simulink model "Model_turn"  (R2024a)
settings: Solver=VariableStepAuto  StartTime=0.0  StopTime=100  MaxStep=0.1  RelTol=1e-3
values from neighbouring files (symbols this model uses):
  c_SMA = 837.36    [params.m]
  Fmax_SMA = 10    [params.m]
  h_SMA = .3    (= 0.3)    [params.m]
  k_gn = m*g/0.01    (= 9810)    [contact3D_params.m]
  k_gt = m*g/0.1    (= 981)    [contact3D_params.m]
  m = 10    [contact3D_params.m]
  m_SMA = 0.0025    [params.m]
  max_SMA_Energy_J = 150    [params.m]
  mu_slide = 0.8    [contact3D_params.m]
  mu_stick = 0.9    [contact3D_params.m]
  n_segs = 10    [params.m]
  PWM_max = 0.35    [params.m]
  R_SMA = .08    (= 0.08)    [params.m]
  r_SMA2limb = 0.009    [params.m]
  swing_angle = swing_angles(i)    [params.m]
  T_amb = 23    [params.m]
  V_0 = 7    [params.m]
  v_gn_max = 0.03    [contact3D_params.m]
  v_gt_max = 0.03    [contact3D_params.m]
  vLimit = 0.01    [contact3D_params.m]
undefined symbols (not defined in the file or in its folder): Newton, Raphson, X, Y, Z
libraries: sm_lib x225, nesl_utility x185, simulink x24, simulink_extras x6
(part 1 of 16)
settings Model: SimulationMode=rapid-accelerator  Creator=lmplo  LastModifiedBy=lmplo

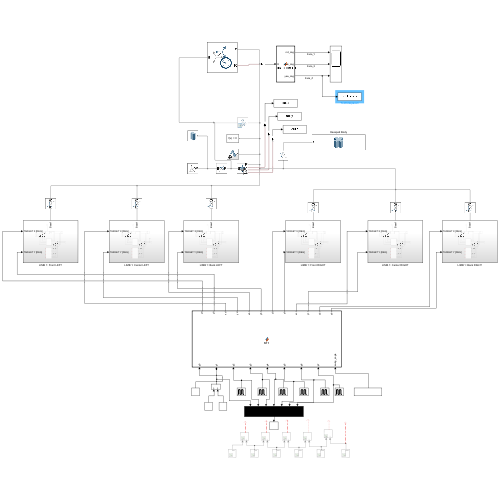
[thumbnail: Simulink's stored preview of the top-level diagram]
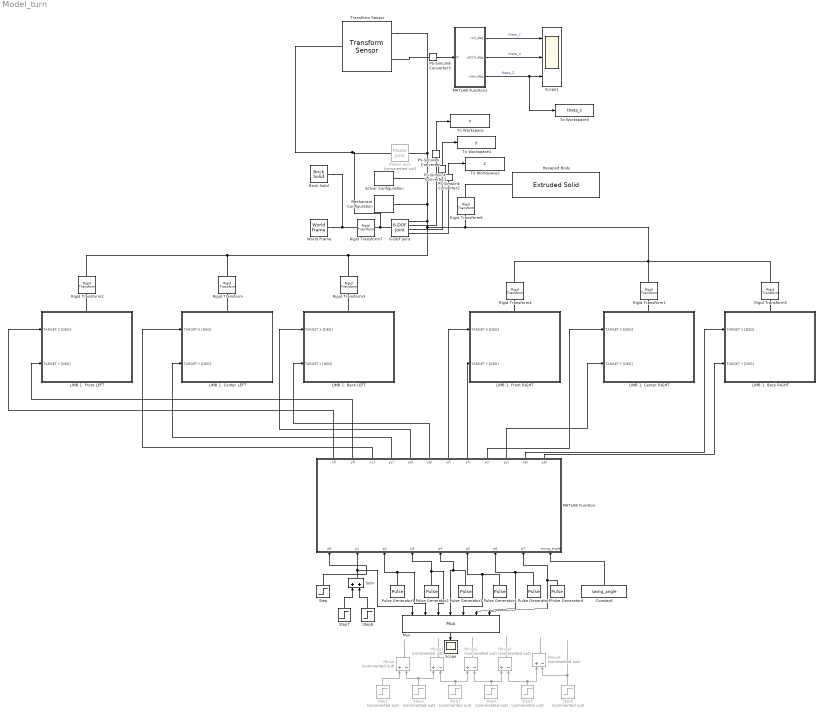
== system Model_turn ==
  6-DOF Joint : sm_lib/Joints/6-DOF Joint  JointMode=Normal  CompositeWrenchDir=FollowerOnBase  CompositeWrenchFrame=BaseFrame  SenseConstraintForce=off  SenseConstraintTorque=off  SenseTotalForce=off  SenseTotalTorque=off  PxPositionTargetSpecify=off  PxPositionTargetPriority=High  PxPositionTargetValue=0  PxPositionTargetValueUnits=m  PxVelocityTargetSpecify=off  PxVelocityTargetPriority=High  PxVelocityTargetValue=0  PxVelocityTargetValueUnits=m/s  PxEquilibriumPosition=0  PxEquilibriumPositionUnits=m  PxSpringStiffness=0  PxSpringStiffnessUnits=N/m  PxDampingCoefficient=0  PxDampingCoefficientUnits=N/(m/s)  PxLowerLimitSpecify=off  PxLowerLimitBound=-1  PxLowerLimitBoundUnits=m  PxLowerLimitStiffness=1e6  PxLowerLimitStiffnessUnits=N/m  PxLowerLimitDamping=1e3  PxLowerLimitDampingUnits=N/(m/s)  PxLowerLimitTransitionRegionWidth=1e-4  PxLowerLimitTransitionRegionWidthUnits=m  PxUpperLimitSpecify=off  PxUpperLimitBound=1  PxUpperLimitBoundUnits=m  PxUpperLimitStiffness=1e6  PxUpperLimitStiffnessUnits=N/m  PxUpperLimitDamping=1e3  PxUpperLimitDampingUnits=N/(m/s)  PxUpperLimitTransitionRegionWidth=1e-4  PxUpperLimitTransitionRegionWidthUnits=m  PxTorqueActuationMode=NoTorque  PxMotionActuationMode=ComputedMotion  PxSensePosition=on  PxSenseVelocity=off  PxSenseAcceleration=off  PxSenseTorqueForce=off  PxSenseLowerLimitTorqueForce=off  PxSenseUpperLimitTorqueForce=off  PyPositionTargetSpecify=off  PyPositionTargetPriority=High  PyPositionTargetValue=0  PyPositionTargetValueUnits=m  PyVelocityTargetSpecify=off  PyVelocityTargetPriority=High  PyVelocityTargetValue=0  PyVelocityTargetValueUnits=m/s  PyEquilibriumPosition=0  PyEquilibriumPositionUnits=m  PySpringStiffness=0  PySpringStiffnessUnits=N/m  PyDampingCoefficient=0  PyDampingCoefficientUnits=N/(m/s)  PyLowerLimitSpecify=off  PyLowerLimitBound=-1  PyLowerLimitBoundUnits=m  PyLowerLimitStiffness=1e6  PyLowerLimitStiffnessUnits=N/m  PyLowerLimitDamping=1e3  PyLowerLimitDampingUnits=N/(m/s)  PyLowerLimitTransitionRegionWidth=1e-4  PyLowerLimitTransitionRegionWidthUnits=m  PyUpperLimitSpecify=off  PyUpperLimitBound=1  PyUpperLimitBoundUnits=m  PyUpperLimitStiffness=1e6  PyUpperLimitStiffnessUnits=N/m  PyUpperLimitDamping=1e3  PyUpperLimitDampingUnits=N/(m/s)  PyUpperLimitTransitionRegionWidth=1e-4  PyUpperLimitTransitionRegionWidthUnits=m  PyTorqueActuationMode=NoTorque  PyMotionActuationMode=ComputedMotion  PySensePosition=on  PySenseVelocity=off  PySenseAcceleration=off  PySenseTorqueForce=off  PySenseLowerLimitTorqueForce=off  PySenseUpperLimitTorqueForce=off  PzPositionTargetSpecify=off  PzPositionTargetPriority=High  PzPositionTargetValue=0  PzPositionTargetValueUnits=m  PzVelocityTargetSpecify=off  PzVelocityTargetPriority=High  PzVelocityTargetValue=0  PzVelocityTargetValueUnits=m/s  PzEquilibriumPosition=0  PzEquilibriumPositionUnits=m  PzSpringStiffness=0  PzSpringStiffnessUnits=N/m  PzDampingCoefficient=0  PzDampingCoefficientUnits=N/(m/s)  PzLowerLimitSpecify=off  PzLowerLimitBound=-1  PzLowerLimitBoundUnits=m  PzLowerLimitStiffness=1e6  PzLowerLimitStiffnessUnits=N/m  PzLowerLimitDamping=1e3  PzLowerLimitDampingUnits=N/(m/s)  PzLowerLimitTransitionRegionWidth=1e-4  PzLowerLimitTransitionRegionWidthUnits=m  PzUpperLimitSpecify=off  PzUpperLimitBound=1  PzUpperLimitBoundUnits=m  PzUpperLimitStiffness=1e6  PzUpperLimitStiffnessUnits=N/m  PzUpperLimitDamping=1e3  PzUpperLimitDampingUnits=N/(m/s)  PzUpperLimitTransitionRegionWidth=1e-4  PzUpperLimitTransitionRegionWidthUnits=m  PzTorqueActuationMode=NoTorque  PzMotionActuationMode=ComputedMotion  PzSensePosition=on  PzSenseVelocity=off  PzSenseAcceleration=off  PzSenseTorqueForce=off  PzSenseLowerLimitTorqueForce=off  PzSenseUpperLimitTorqueForce=off  SphPositionTargetSpecify=off  SphPositionTargetPriority=High  SphPositionTargetRotationMethod=None  SphPositionTargetFollAlignAxisA=+X  SphPositionTargetBaseAlignAxisA=+Y  SphPositionTargetFollAlignAxisB=+Y  SphPositionTargetBaseAlignAxisB=+Z  SphPositionTargetRotationStandardAxis=+Z  SphPositionTargetRotationAngle=0  SphPositionTargetRotationAngleUnits=deg  SphPositionTargetRotationArbitraryAxis=[0 0 1]  SphPositionTargetRotationSequenceAxes=FollowerAxes  SphPositionTargetRotationSequence=XYX  SphPositionTargetRotationSequenceAngles=[0 0 0]  SphPositionTargetRotationSequenceAnglesUnits=deg  SphPositionTargetRotationMatrix=[1 0 0;0 1 0;0 0 1]  SphPositionTargetQuaternion=[1 0 0 0]  SphVelocityTargetSpecify=off  SphVelocityTargetPriority=High  SphVelocityTargetValue=[0 0 0]  SphVelocityTargetValueUnits=deg/s  SphVelocityTargetInFollowerFrame=on  SphEqPosRotationMethod=None  SphEqPosFollAlignAxisA=+X  SphEqPosBaseAlignAxisA=+Y  SphEqPosFollAlignAxisB=+Y  SphEqPosBaseAlignAxisB=+Z  SphEqPosRotationStandardAxis=+Z  SphEqPosRotationAngle=0  SphEqPosRotationAngleUnits=deg  SphEqPosRotationArbitraryAxis=[0 0 1]  SphEqPosRotationSequenceAxes=FollowerAxes  SphEqPosRotationSequence=XYX  SphEqPosRotationSequenceAngles=[0 0 0]  SphEqPosRotationSequenceAnglesUnits=deg  SphEqPosRotationMatrix=[1 0 0;0 1 0;0 0 1]  SphEqPosQuaternion=[1 0 0 0]  SphSpringStiffness=0  SphSpringStiffnessUnits=N*m/deg  SphDampingCoefficient=0  SphDampingCoefficientUnits=N*m/(deg/s)  SphLowerLimitSpecify=off  SphLowerLimitBound=15  SphLowerLimitBoundUnits=deg  SphLowerLimitStiffness=1e4  SphLowerLimitStiffnessUnits=N*m/deg  SphLowerLimitDamping=10  SphLowerLimitDampingUnits=N*m/(deg/s)  SphLowerLimitTransitionRegionWidth=0.1  SphLowerLimitTransitionRegionWidthUnits=deg  SphUpperLimitSpecify=off  SphUpperLimitBound=45  SphUpperLimitBoundUnits=deg  SphUpperLimitStiffness=1e4  SphUpperLimitStiffnessUnits=N*m/deg  SphUpperLimitDamping=10  SphUpperLimitDampingUnits=N*m/(deg/s)  SphUpperLimitTransitionRegionWidth=0.1  SphUpperLimitTransitionRegionWidthUnits=deg  SphTorqueActuationMode=NoTorque  SphActuateTorqueX=off  SphActuateTorqueY=off  SphActuateTorqueZ=off  SphActuateTorque=off  SphActuationFrame=BaseFrame  SphSensePosition=off  SphSenseVelocityX=off  SphSenseVelocityY=off  SphSenseVelocityZ=off  SphSenseVelocity=off  SphSenseAccelerationX=off  SphSenseAccelerationY=off  SphSenseAccelerationZ=off  SphSenseAcceleration=off  SphSenseLowerLimitTorqueMag=off  SphSenseUpperLimitTorqueMag=off  SphSensingFrame=BaseFrame
  Brick Solid : sm_lib/Body Elements/Brick Solid  BrickDimensions=[10 10 0.001]  BrickDimensionsUnits=m  ExportEntireGeometry=off  InertiaType=CalculateFromGeometry  BasedOnType=Density  Density=1000  DensityUnits=kg/m^3  Mass=1  MassUnits=kg  CenterOfMass=[0 0 0]  CenterOfMassUnits=m  MomentsOfInertia=[1 1 1]  MomentsOfInertiaUnits=kg*m^2  ProductsOfInertia=[0 0 0]  ProductsOfInertiaUnits=kg*m^2  GraphicType=FromGeometry  MarkerShape=Sphere  MarkerSize=10  GraphicVisPropType=SimpleVisualProperties  GraphicDiffuseColor=[0.4 0.2 0.0]  GraphicOpacity=1  GraphicSpecularColor=[0.5 0.5 0.5 1.0]  GraphicAmbientColor=[0.15 0.15 0.15 1.0]  GraphicEmissiveColor=[0.0 0.0 0.0 1.0]  GraphicShininess=75  DoExposeReferenceFrame=on  SerializedFrames=<Frames/>
  Constant : Constant  Value=swing_angle
  Hexapod Body : sm_lib/Body Elements/Extruded Solid  ExtrusionType=General  PolygonNumSides=6  PolygonOuterRadius=.1  PolygonOuterRadiusUnits=m  ExportEntireGeometry=off  ExtrusionCrossSection=[-.1 0; -.05 -.07; .05 -.07; .1 0; .05 .07; -.05 .07]  ExtrusionCrossSectionUnits=m  ExportConvexHullGeometry=off  ExtrusionLength=.05  ExtrusionLengthUnits=m  InertiaType=CalculateFromGeometry  BasedOnType=Density  Density=10  DensityUnits=kg/m^3  Mass=1  MassUnits=kg  CenterOfMass=[0 0 0]  CenterOfMassUnits=m  MomentsOfInertia=[1 1 1]  MomentsOfInertiaUnits=kg*m^2  ProductsOfInertia=[0 0 0]  ProductsOfInertiaUnits=kg*m^2  GraphicType=FromGeometry  MarkerShape=Sphere  MarkerSize=10  GraphicVisPropType=SimpleVisualProperties  GraphicDiffuseColor=[0.5 0.5 0.5]  GraphicOpacity=1  GraphicSpecularColor=[0.5 0.5 0.5 1.0]  GraphicAmbientColor=[0.15 0.15 0.15 1.0]  GraphicEmissiveColor=[0.0 0.0 0.0 1.0]  GraphicShininess=75  DoExposeReferenceFrame=on  SerializedFrames=<Frames/>
  LIMB 1: Back LEFT : Subsystem
      settings: PortSchema="{\"entries\":[{\"content\":{\"sides\":[{\"content\":{\"connectorIds\":[\"In1\",\"In2\"]},\"type\":\"ConnectorPlacement.EquallySpacedRectSide\",\"uuid\":\"dac3a422-23dc-41de-9456-f1b703ee7ea4\"},{\"content\":{\"side\":\"RIGHT\"},\"type\":\"ConnectorPlacement.EquallySpacedRectSide\",\"uuid\":\"acd4b41e-2563-470e-afc8-f7cd5e457540\"},{\"content\":{\"connectorIds\":[\"LConn1\"],\"side\":\"TOP\"},\"type\":\"ConnectorPlacement.EquallySpacedRectSide\",\"uuid\":\"2403ebe1-3ea7-4eb6-be2b-197ca3d8e68e\"}]},\"type\":\"ConnectorPlacement.EquallySpacedConnector\",\"uuid\":\"537b2e86-94c9-41ef-b748-fab54b193b4a\"}],\"packageUris\":[\"http://schema.mathworks.com/mf0/Connector/R2020b\"],\"version\":\"1.0\"}"
  LIMB 1: Back RIGHT : Subsystem
      settings: PortSchema="{\"entries\":[{\"content\":{\"sides\":[{\"content\":{\"connectorIds\":[\"In1\",\"In2\"]},\"type\":\"ConnectorPlacement.EquallySpacedRectSide\",\"uuid\":\"dac3a422-23dc-41de-9456-f1b703ee7ea4\"},{\"content\":{\"side\":\"RIGHT\"},\"type\":\"ConnectorPlacement.EquallySpacedRectSide\",\"uuid\":\"acd4b41e-2563-470e-afc8-f7cd5e457540\"},{\"content\":{\"connectorIds\":[\"LConn1\"],\"side\":\"TOP\"},\"type\":\"ConnectorPlacement.EquallySpacedRectSide\",\"uuid\":\"2403ebe1-3ea7-4eb6-be2b-197ca3d8e68e\"}]},\"type\":\"ConnectorPlacement.EquallySpacedConnector\",\"uuid\":\"537b2e86-94c9-41ef-b748-fab54b193b4a\"}],\"packageUris\":[\"http://schema.mathworks.com/mf0/Connector/R2020b\"],\"version\":\"1.0\"}"
  LIMB 1: Center LEFT : Subsystem
      settings: PortSchema="{\"entries\":[{\"content\":{\"sides\":[{\"content\":{\"connectorIds\":[\"In1\",\"In2\"]},\"type\":\"ConnectorPlacement.EquallySpacedRectSide\",\"uuid\":\"dac3a422-23dc-41de-9456-f1b703ee7ea4\"},{\"content\":{\"side\":\"RIGHT\"},\"type\":\"ConnectorPlacement.EquallySpacedRectSide\",\"uuid\":\"acd4b41e-2563-470e-afc8-f7cd5e457540\"},{\"content\":{\"connectorIds\":[\"LConn1\"],\"side\":\"TOP\"},\"type\":\"ConnectorPlacement.EquallySpacedRectSide\",\"uuid\":\"2403ebe1-3ea7-4eb6-be2b-197ca3d8e68e\"}]},\"type\":\"ConnectorPlacement.EquallySpacedConnector\",\"uuid\":\"537b2e86-94c9-41ef-b748-fab54b193b4a\"}],\"packageUris\":[\"http://schema.mathworks.com/mf0/Connector/R2020b\"],\"version\":\"1.0\"}"
  LIMB 1: Center RIGHT : Subsystem
      settings: PortSchema="{\"entries\":[{\"content\":{\"sides\":[{\"content\":{\"connectorIds\":[\"In1\",\"In2\"]},\"type\":\"ConnectorPlacement.EquallySpacedRectSide\",\"uuid\":\"dac3a422-23dc-41de-9456-f1b703ee7ea4\"},{\"content\":{\"side\":\"RIGHT\"},\"type\":\"ConnectorPlacement.EquallySpacedRectSide\",\"uuid\":\"acd4b41e-2563-470e-afc8-f7cd5e457540\"},{\"content\":{\"connectorIds\":[\"LConn1\"],\"side\":\"TOP\"},\"type\":\"ConnectorPlacement.EquallySpacedRectSide\",\"uuid\":\"2403ebe1-3ea7-4eb6-be2b-197ca3d8e68e\"}]},\"type\":\"ConnectorPlacement.EquallySpacedConnector\",\"uuid\":\"537b2e86-94c9-41ef-b748-fab54b193b4a\"}],\"packageUris\":[\"http://schema.mathworks.com/mf0/Connector/R2020b\"],\"version\":\"1.0\"}"
  LIMB 1: Front LEFT : Subsystem
      settings: PortSchema="{\"entries\":[{\"content\":{\"sides\":[{\"content\":{\"connectorIds\":[\"In1\",\"In2\"]},\"type\":\"ConnectorPlacement.EquallySpacedRectSide\",\"uuid\":\"dac3a422-23dc-41de-9456-f1b703ee7ea4\"},{\"content\":{\"side\":\"RIGHT\"},\"type\":\"ConnectorPlacement.EquallySpacedRectSide\",\"uuid\":\"acd4b41e-2563-470e-afc8-f7cd5e457540\"},{\"content\":{\"connectorIds\":[\"LConn1\"],\"side\":\"TOP\"},\"type\":\"ConnectorPlacement.EquallySpacedRectSide\",\"uuid\":\"2403ebe1-3ea7-4eb6-be2b-197ca3d8e68e\"}]},\"type\":\"ConnectorPlacement.EquallySpacedConnector\",\"uuid\":\"537b2e86-94c9-41ef-b748-fab54b193b4a\"}],\"packageUris\":[\"http://schema.mathworks.com/mf0/Connector/R2020b\"],\"version\":\"1.0\"}"
  LIMB 1: Front RIGHT : Subsystem
      settings: PortSchema="{\"entries\":[{\"content\":{\"sides\":[{\"content\":{\"connectorIds\":[\"In1\",\"In2\"]},\"type\":\"ConnectorPlacement.EquallySpacedRectSide\",\"uuid\":\"dac3a422-23dc-41de-9456-f1b703ee7ea4\"},{\"content\":{\"side\":\"RIGHT\"},\"type\":\"ConnectorPlacement.EquallySpacedRectSide\",\"uuid\":\"acd4b41e-2563-470e-afc8-f7cd5e457540\"},{\"content\":{\"connectorIds\":[\"LConn1\"],\"side\":\"TOP\"},\"type\":\"ConnectorPlacement.EquallySpacedRectSide\",\"uuid\":\"2403ebe1-3ea7-4eb6-be2b-197ca3d8e68e\"}]},\"type\":\"ConnectorPlacement.EquallySpacedConnector\",\"uuid\":\"537b2e86-94c9-41ef-b748-fab54b193b4a\"}],\"packageUris\":[\"http://schema.mathworks.com/mf0/Connector/R2020b\"],\"version\":\"1.0\"}"
  MATLAB Function : MATLAB Function  TreatAsAtomicUnit=on
  MATLAB Function1 : MATLAB Function  TreatAsAtomicUnit=on
  Mechanism Configuration : sm_lib/Utilities/Mechanism Configuration  UniformGravity=Constant  GravityVector=[0 0 -9.80665]  GravityVectorUnits=m/s^2  LinearizationDelta=0.001  JointModeTransitionNonlinearIterations=2
  Minus{,1..4} (5 alike) : Sum  Commented=on  Inputs=+-
  Mux : Mux  Inputs=7
  PS-Simulink Converter{,1..3} (4 alike) : nesl_utility/PS-Simulink Converter  PhysicalDomain=network_engine_domain  SubClassName=ps_output  LeftPortType=input  RightPortType=output  PseudoPeriodic=off  Frequencies=[]  VectorFormat=inherit  Unit=inherit  AffineConversion=off
  Planar Joint : sm_lib/Joints/Planar Joint  Commented=on  JointMode=Normal  CompositeWrenchDir=FollowerOnBase  CompositeWrenchFrame=BaseFrame  SenseConstraintForce=off  SenseConstraintTorque=off  SenseTotalForce=off  SenseTotalTorque=off  PxPositionTargetSpecify=off  PxPositionTargetPriority=High  PxPositionTargetValue=0  PxPositionTargetValueUnits=m  PxVelocityTargetSpecify=off  PxVelocityTargetPriority=High  PxVelocityTargetValue=0  PxVelocityTargetValueUnits=m/s  PxEquilibriumPosition=0  PxEquilibriumPositionUnits=m  PxSpringStiffness=0  PxSpringStiffnessUnits=N/m  PxDampingCoefficient=0  PxDampingCoefficientUnits=N/(m/s)  PxLowerLimitSpecify=off  PxLowerLimitBound=-1  PxLowerLimitBoundUnits=m  PxLowerLimitStiffness=1e6  PxLowerLimitStiffnessUnits=N/m  PxLowerLimitDamping=1e3  PxLowerLimitDampingUnits=N/(m/s)  PxLowerLimitTransitionRegionWidth=1e-4  PxLowerLimitTransitionRegionWidthUnits=m  PxUpperLimitSpecify=off  PxUpperLimitBound=1  PxUpperLimitBoundUnits=m  PxUpperLimitStiffness=1e6  PxUpperLimitStiffnessUnits=N/m  PxUpperLimitDamping=1e3  PxUpperLimitDampingUnits=N/(m/s)  PxUpperLimitTransitionRegionWidth=1e-4  PxUpperLimitTransitionRegionWidthUnits=m  PxTorqueActuationMode=NoTorque  PxMotionActuationMode=ComputedMotion  PxSensePosition=off  PxSenseVelocity=off  PxSenseAcceleration=off  PxSenseTorqueForce=off  PxSenseLowerLimitTorqueForce=off  PxSenseUpperLimitTorqueForce=off  PyPositionTargetSpecify=off  PyPositionTargetPriority=High  PyPositionTargetValue=0  PyPositionTargetValueUnits=m  PyVelocityTargetSpecify=off  PyVelocityTargetPriority=High  PyVelocityTargetValue=0  PyVelocityTargetValueUnits=m/s  PyEquilibriumPosition=0  PyEquilibriumPositionUnits=m  PySpringStiffness=0  PySpringStiffnessUnits=N/m  PyDampingCoefficient=0  PyDampingCoefficientUnits=N/(m/s)  PyLowerLimitSpecify=off  PyLowerLimitBound=-1  PyLowerLimitBoundUnits=m  PyLowerLimitStiffness=1e6  PyLowerLimitStiffnessUnits=N/m  PyLowerLimitDamping=1e3  PyLowerLimitDampingUnits=N/(m/s)  PyLowerLimitTransitionRegionWidth=1e-4  PyLowerLimitTransitionRegionWidthUnits=m  PyUpperLimitSpecify=off  PyUpperLimitBound=1  PyUpperLimitBoundUnits=m  PyUpperLimitStiffness=1e6  PyUpperLimitStiffnessUnits=N/m  PyUpperLimitDamping=1e3  PyUpperLimitDampingUnits=N/(m/s)  PyUpperLimitTransitionRegionWidth=1e-4  PyUpperLimitTransitionRegionWidthUnits=m  PyTorqueActuationMode=NoTorque  PyMotionActuationMode=ComputedMotion  PySensePosition=off  PySenseVelocity=off  PySenseAcceleration=off  PySenseTorqueForce=off  PySenseLowerLimitTorqueForce=off  PySenseUpperLimitTorqueForce=off  RzPositionTargetSpecify=off  RzPositionTargetPriority=High  RzPositionTargetValue=0  RzPositionTargetValueUnits=deg  RzVelocityTargetSpecify=off  RzVelocityTargetPriority=High  RzVelocityTargetValue=0  RzVelocityTargetValueUnits=deg/s  RzEquilibriumPosition=0  RzEquilibriumPositionUnits=deg  RzSpringStiffness=0  RzSpringStiffnessUnits=N*m/deg  RzDampingCoefficient=0  RzDampingCoefficientUnits=N*m/(deg/s)  RzLowerLimitSpecify=off  RzLowerLimitBound=-90  RzLowerLimitBoundUnits=deg  RzLowerLimitStiffness=1e4  RzLowerLimitStiffnessUnits=N*m/deg  RzLowerLimitDamping=10  RzLowerLimitDampingUnits=N*m/(deg/s)  RzLowerLimitTransitionRegionWidth=0.1  RzLowerLimitTransitionRegionWidthUnits=deg  RzUpperLimitSpecify=off  RzUpperLimitBound=90  RzUpperLimitBoundUnits=deg  RzUpperLimitStiffness=1e4  RzUpperLimitStiffnessUnits=N*m/deg  RzUpperLimitDamping=10  RzUpperLimitDampingUnits=N*m/(deg/s)  RzUpperLimitTransitionRegionWidth=0.1  RzUpperLimitTransitionRegionWidthUnits=deg  RzTorqueActuationMode=NoTorque  RzMotionActuationMode=ComputedMotion  RzSensePosition=off  RzSenseVelocity=off  RzSenseAcceleration=off  RzSenseTorqueForce=off  RzSenseLowerLimitTorqueForce=off  RzSenseUpperLimitTorqueForce=off
  Pulse Generator1 : DiscretePulseGenerator  PulseType=Time based  Period=30  PulseWidth=16  PhaseDelay=10
  Pulse Generator2 : DiscretePulseGenerator  PulseType=Time based  Period=30  PulseWidth=16  PhaseDelay=15
  Pulse Generator3 : DiscretePulseGenerator  PulseType=Time based  Period=30  PulseWidth=16  PhaseDelay=20
  Pulse Generator4 : DiscretePulseGenerator  PulseType=Time based  Period=30  PulseWidth=16  PhaseDelay=25
  Pulse Generator5 : DiscretePulseGenerator  PulseType=Time based  Period=30  PulseWidth=16  PhaseDelay=30
  Pulse Generator6 : DiscretePulseGenerator  PulseType=Time based  Period=30  PulseWidth=16  PhaseDelay=35
  Rigid Transform : sm_lib/Frames and Transforms/Rigid Transform  RotationMethod=StandardAxis  FollAlignAxisA=+X  BaseAlignAxisA=+Y  FollAlignAxisB=+Y  BaseAlignAxisB=+Z  RotationStandardAxis=+Y  RotationAngle=30  RotationAngleUnits=deg  RotationArbitraryAxis=[0 0 1]  RotationSequenceAxes=FollowerAxes  RotationSequence=XYX  RotationSequenceAngles=[0 0 0]  RotationSequenceAnglesUnits=deg  RotationMatrix=[1 0 0;0 1 0;0 0 1]  Quaternion=[1 0 0 0]  TranslationMethod=Cartesian  TranslationCartesianOffset=[-0.1 0 0]  TranslationCartesianOffsetUnits=m  TranslationStandardAxis=+Z  TranslationStandardOffset=0  TranslationStandardOffsetUnits=m  TranslationROffset=0  TranslationROffsetUnits=m  TranslationThetaOffset=0  TranslationThetaOffsetUnits=deg  TranslationZOffset=0  TranslationZOffsetUnits=m
  Rigid Transform1 : sm_lib/Frames and Transforms/Rigid Transform  RotationMethod=StandardAxis  FollAlignAxisA=+X  BaseAlignAxisA=+Y  FollAlignAxisB=+Y  BaseAlignAxisB=+Z  RotationStandardAxis=+Y  RotationAngle=-30  RotationAngleUnits=deg  RotationArbitraryAxis=[0 0 1]  RotationSequenceAxes=FollowerAxes  RotationSequence=XYX  RotationSequenceAngles=[0 0 0]  RotationSequenceAnglesUnits=deg  RotationMatrix=[1 0 0;0 1 0;0 0 1]  Quaternion=[1 0 0 0]  TranslationMethod=Cartesian  TranslationCartesianOffset=[0.1 0 0]  TranslationCartesianOffsetUnits=m  TranslationStandardAxis=+Z  TranslationStandardOffset=0  TranslationStandardOffsetUnits=m  TranslationROffset=0  TranslationROffsetUnits=m  TranslationThetaOffset=0  TranslationThetaOffsetUnits=deg  TranslationZOffset=0  TranslationZOffsetUnits=m
  Rigid Transform2 : sm_lib/Frames and Transforms/Rigid Transform  RotationMethod=StandardAxis  FollAlignAxisA=+X  BaseAlignAxisA=+Y  FollAlignAxisB=+Y  BaseAlignAxisB=+Z  RotationStandardAxis=+Y  RotationAngle=30  RotationAngleUnits=deg  RotationArbitraryAxis=[0 0 1]  RotationSequenceAxes=BaseAxes  RotationSequence=XYZ  RotationSequenceAngles=[0 0 0]  RotationSequenceAnglesUnits=deg  RotationMatrix=[1 0 0;0 1 0;0 0 1]  Quaternion=[1 0 0 0]  TranslationMethod=Cartesian  TranslationCartesianOffset=[-0.05 0.07 0]  TranslationCartesianOffsetUnits=m  TranslationStandardAxis=+Z  TranslationStandardOffset=0  TranslationStandardOffsetUnits=m  TranslationROffset=0  TranslationROffsetUnits=m  TranslationThetaOffset=0  TranslationThetaOffsetUnits=deg  TranslationZOffset=0  TranslationZOffsetUnits=m
  Rigid Transform3 : sm_lib/Frames and Transforms/Rigid Transform  RotationMethod=StandardAxis  FollAlignAxisA=+X  BaseAlignAxisA=+Y  FollAlignAxisB=+Y  BaseAlignAxisB=+Z  RotationStandardAxis=+Y  RotationAngle=30  RotationAngleUnits=deg  RotationArbitraryAxis=[0 0 1]  RotationSequenceAxes=FollowerAxes  RotationSequence=XYX  RotationSequenceAngles=[0 0 0]  RotationSequenceAnglesUnits=deg  RotationMatrix=[1 0 0;0 1 0;0 0 1]  Quaternion=[1 0 0 0]  TranslationMethod=Cartesian  TranslationCartesianOffset=[-0.05 -0.07 0]  TranslationCartesianOffsetUnits=m  TranslationStandardAxis=+Z  TranslationStandardOffset=0  TranslationStandardOffsetUnits=m  TranslationROffset=0  TranslationROffsetUnits=m  TranslationThetaOffset=0  TranslationThetaOffsetUnits=deg  TranslationZOffset=0  TranslationZOffsetUnits=m
  Rigid Transform4 : sm_lib/Frames and Transforms/Rigid Transform  RotationMethod=StandardAxis  FollAlignAxisA=+X  BaseAlignAxisA=+Y  FollAlignAxisB=+Y  BaseAlignAxisB=+Z  RotationStandardAxis=+Y  RotationAngle=-30  RotationAngleUnits=deg  RotationArbitraryAxis=[0 0 1]  RotationSequenceAxes=BaseAxes  RotationSequence=XYZ  RotationSequenceAngles=[0 0 0]  RotationSequenceAnglesUnits=deg  RotationMatrix=[1 0 0;0 1 0;0 0 1]  Quaternion=[1 0 0 0]  TranslationMethod=Cartesian  TranslationCartesianOffset=[0.05 0.07 0]  TranslationCartesianOffsetUnits=m  TranslationStandardAxis=+Z  TranslationStandardOffset=0  TranslationStandardOffsetUnits=m  TranslationROffset=0  TranslationROffsetUnits=m  TranslationThetaOffset=0  TranslationThetaOffsetUnits=deg  TranslationZOffset=0  TranslationZOffsetUnits=m
  Rigid Transform5 : sm_lib/Frames and Transforms/Rigid Transform  RotationMethod=StandardAxis  FollAlignAxisA=+X  BaseAlignAxisA=+Y  FollAlignAxisB=+Y  BaseAlignAxisB=+Z  RotationStandardAxis=+Y  RotationAngle=-30  RotationAngleUnits=deg  RotationArbitraryAxis=[0 0 1]  RotationSequenceAxes=FollowerAxes  RotationSequence=XYX  RotationSequenceAngles=[0 0 0]  RotationSequenceAnglesUnits=deg  RotationMatrix=[1 0 0;0 1 0;0 0 1]  Quaternion=[1 0 0 0]  TranslationMethod=Cartesian  TranslationCartesianOffset=[0.05 -0.07 0]  TranslationCartesianOffsetUnits=m  TranslationStandardAxis=+Z  TranslationStandardOffset=0  TranslationStandardOffsetUnits=m  TranslationROffset=0  TranslationROffsetUnits=m  TranslationThetaOffset=0  TranslationThetaOffsetUnits=deg  TranslationZOffset=0  TranslationZOffsetUnits=m
  Rigid Transform6 : sm_lib/Frames and Transforms/Rigid Transform  RotationMethod=None  FollAlignAxisA=+X  BaseAlignAxisA=+Y  FollAlignAxisB=+Y  BaseAlignAxisB=+Z  RotationStandardAxis=+Z  RotationAngle=0  RotationAngleUnits=deg  RotationArbitraryAxis=[0 0 1]  RotationSequenceAxes=FollowerAxes  RotationSequence=XYX  RotationSequenceAngles=[0 0 0]  RotationSequenceAnglesUnits=deg  RotationMatrix=[1 0 0;0 1 0;0 0 1]  Quaternion=[1 0 0 0]  TranslationMethod=Cartesian  TranslationCartesianOffset=[0 0 0.02]  TranslationCartesianOffsetUnits=m  TranslationStandardAxis=+Z  TranslationStandardOffset=0  TranslationStandardOffsetUnits=m  TranslationROffset=0  TranslationROffsetUnits=m  TranslationThetaOffset=0  TranslationThetaOffsetUnits=deg  TranslationZOffset=0  TranslationZOffsetUnits=m
  Rigid Transform7 : sm_lib/Frames and Transforms/Rigid Transform  RotationMethod=StandardAxis  FollAlignAxisA=+X  BaseAlignAxisA=+Y  FollAlignAxisB=+Y  BaseAlignAxisB=+Z  RotationStandardAxis=+Y  RotationAngle=0  RotationAngleUnits=deg  RotationArbitraryAxis=[0 0 1]  RotationSequenceAxes=FollowerAxes  RotationSequence=XYX  RotationSequenceAngles=[0 0 0]  RotationSequenceAnglesUnits=deg  RotationMatrix=[1 0 0;0 1 0;0 0 1]  Quaternion=[1 0 0 0]  TranslationMethod=Cartesian  TranslationCartesianOffset=[0 0 0.87]  TranslationCartesianOffsetUnits=m  TranslationStandardAxis=+Z  TranslationStandardOffset=0  TranslationStandardOffsetUnits=m  TranslationROffset=0  TranslationROffsetUnits=m  TranslationThetaOffset=0  TranslationThetaOffsetUnits=deg  TranslationZOffset=0  TranslationZOffsetUnits=m
  Scope : Scope
  Scope1 : Scope  NumInputPorts=3
  Solver Configuration : nesl_utility/Solver Configuration  PhysicalDomain=network_engine_domain  SubClassName=solver  LeftPortType=input  RightPortType=generic  Tones=[]  Harmonics=[]  SimulateNoise=off  Profile=off  UseLocalSampling=off  EnableSwitchedLinearOptims=on  FrequencyDomain=off  UseCCode=off  RelTol=0.001  AbsTol=0.001  MinStep=1e-09  ToWorkspace=off  RevertToSquareIcSolve=off  NumHomotopyIterations=100  PhasorMode=off  PhasorModeNumHarmonics=1  ConsistencySolver=NEWTON_XTOL_AFTER_FTOL  IndexReductionMethod=DerivativeReplacement  DoDC=off  ResidualTolerance=1e-09  ConsistencyTolSource=GLOBAL  ConsistencyAbsTol=0.001  ConsistencyRelTol=0.001  ConsistencyTolFactor=0.001  UseLocalSolver=off  LocalSolverChoice=NE_BACKWARD_EULER_ADVANCER  ResolveIndetEquations=on  FunctionEvalNumThread=1  LocalSolverSampleTime=0.001  DoFixedCost=off  MaxNonlinIter=3  MaxModeIter=2  ComputeImpulses=off  ImpulseIterations=2  LinearAlgebra=auto  LinearAlgebraNumThread=0  EquationFormulation=NE_TIME_EF  DelaysMemoryBudget=1024  AutomaticFiltering=on  FilteringTimeConstant=0.001  PartitionStorageMethod=AS_NEEDED  PartitionMemoryBudget=1024  PartitionMethod=ROBUST  MultibodyUseLocalSolver=off  MultibodyLocalSolverChoice=ODE1  MultibodyLocalSolverSampleTime=0.001
  Step : Step  Time=5  Before=1  After=0  SampleTime=0
  Step1 : Step  Commented=on  Time=5  SampleTime=0
  Step2 : Step  Commented=on  Time=10  SampleTime=0
  Step3 : Step  Commented=on  Time=15  SampleTime=0
  Step4 : Step  Commented=on  Time=20  SampleTime=0
  Step5 : Step  Commented=on  Time=25  SampleTime=0
  Step6 : Step  Commented=on  Time=30  SampleTime=0
  Step7 : Step  Time=5  SampleTime=0
  Step8 : Step  Time=10  After=-1  SampleTime=0
  Sum : Sum
  To Workspace : ToWorkspace  VariableName=x  SaveFormat=Timeseries  SampleTime=-1
  To Workspace1 : ToWorkspace  VariableName=y  SaveFormat=Timeseries  SampleTime=-1
  To Workspace2 : ToWorkspace  VariableName=z  SaveFormat=Timeseries  SampleTime=-1
  To Workspace3 : ToWorkspace  VariableName=theta_z  SaveFormat=Timeseries  SampleTime=-1
  Transform Sensor : sm_lib/Frames and Transforms/Transform Sensor  MeasurementFrame=NonRotatingBase  RotationSequence=XYZ  SenseAngle=off  SenseAxis=off  SenseQ=off  SenseR=on  SenseRotationSequence=off  SenseOmegaX=off  SenseOmegaY=off  SenseOmegaZ=off  SenseOmega=off  SenseQDot=off  SenseRDot=off  SenseRotationSequenceDot=off  SenseAlphaX=off  SenseAlphaY=off  SenseAlphaZ=off  SenseAlpha=off  SenseQDDot=off  SenseRDDot=off  SenseX=off  SenseY=off  SenseZ=off  SenseXYZ=off  SenseRad=off  SenseAzim=off  SenseDist=off  SenseInc=off  SenseXDot=off  SenseYDot=off  SenseZDot=off  SenseXYZDot=off  SenseRadDot=off  SenseAzimDot=off  SenseDistDot=off  SenseIncDot=off  SenseXDDot=off  SenseYDDot=off  SenseZDDot=off  SenseXYZDDot=off  SenseRadDDot=off  SenseAzimDDot=off  SenseDistDDot=off  SenseIncDDot=off
  World Frame : sm_lib/Frames and Transforms/World Frame
  wires:
  MATLAB Function/1(xfl) -> LIMB 1: Front LEFT/1(TARGET X [DEG])
  MATLAB Function/2(yfl) -> LIMB 1: Front LEFT/2(TARGET Y [DEG])
  MATLAB Function/3(xcl) -> LIMB 1: Center LEFT/1(TARGET X [DEG])
  MATLAB Function/4(ycl) -> LIMB 1: Center LEFT/2(TARGET Y [DEG])
  MATLAB Function/5(xbl) -> LIMB 1: Back LEFT/1(TARGET X [DEG])
  MATLAB Function/6(ybl) -> LIMB 1: Back LEFT/2(TARGET Y [DEG])
  MATLAB Function/7(xfr) -> LIMB 1: Front RIGHT/1(TARGET X [DEG])
  MATLAB Function/8(yfr) -> LIMB 1: Front RIGHT/2(TARGET Y [DEG])
  MATLAB Function/9(xcr) -> LIMB 1: Center RIGHT/1(TARGET X [DEG])
  MATLAB Function/10(ycr) -> LIMB 1: Center RIGHT/2(TARGET Y [DEG])
  MATLAB Function/11(xbr) -> LIMB 1: Back RIGHT/1(TARGET X [DEG])
  MATLAB Function/12(ybr) -> LIMB 1: Back RIGHT/2(TARGET Y [DEG])
  Step4/1 -> Minus3/1, Minus2/2
  Minus/1 -> ?
  Step1/1 -> Minus/1
  Step2/1 -> Minus1/1, Minus/2
  Minus1/1 -> ?
  Step3/1 -> Minus2/1, Minus1/2
  Minus2/1 -> ?
  Step/1 -> MATLAB Function/1(p0)
  Minus3/1 -> ?
  Step5/1 -> Minus3/2, Minus4/1
  Minus4/1 -> ?
  Step6/1 -> Minus4/2
  Pulse Generator1/1 -> Mux/2, MATLAB Function/3(p2)
  Pulse Generator2/1 -> Mux/3, MATLAB Function/4(p3)
  Pulse Generator3/1 -> Mux/4, MATLAB Function/5(p4)
  Pulse Generator4/1 -> Mux/5, MATLAB Function/6(p5)
  Pulse Generator5/1 -> Mux/6, MATLAB Function/7(p6)
  Mux/1 -> Scope/1
  Pulse Generator6/1 -> Mux/7, MATLAB Function/8(p7)
  Sum/1 -> Mux/1, MATLAB Function/2(p1)
  Step7/1 -> Sum/1
  Step8/1 -> Sum/2
  Constant/1 -> MATLAB Function/9(swing_angle)
  PS-Simulink Converter/1 -> To Workspace/1
  PS-Simulink Converter1/1 -> To Workspace1/1
  PS-Simulink Converter2/1 -> To Workspace2/1
  MATLAB Function1/2(pitch_deg) -> Scope1/2  "theta_X"
  PS-Simulink Converter3/1 -> MATLAB Function1/1(R)
  MATLAB Function1/3(yaw_deg) -> To Workspace3/1, Scope1/3  "theta_Z"
  MATLAB Function1/1(roll_deg) -> Scope1/1  "theta_Y"
  connections:
  Rigid Transform/RConn1 -- LIMB 1: Center LEFT/LConn1
  Rigid Transform2/RConn1 -- LIMB 1: Front LEFT/LConn1
  Rigid Transform3/RConn1 -- LIMB 1: Back LEFT/LConn1
  Planar Joint/RConn1 -- Transform Sensor/RConn1 -- Solver Configuration/RConn1 -- Mechanism Configuration/RConn1 -- Rigid Transform5/LConn1 -- Rigid Transform1/LConn1 -- Rigid Transform4/LConn1 -- Rigid Transform6/LConn1 -- Rigid Transform2/LConn1 -- Rigid Transform/LConn1 -- Rigid Transform3/LConn1 -- 6-DOF Joint/RConn1
  Rigid Transform5/RConn1 -- LIMB 1: Back RIGHT/LConn1
  Rigid Transform1/RConn1 -- LIMB 1: Center RIGHT/LConn1
  Rigid Transform4/RConn1 -- LIMB 1: Front RIGHT/LConn1
  Hexapod Body/RConn1 -- Rigid Transform6/RConn1
  World Frame/RConn1 -- Brick Solid/RConn1 -- Rigid Transform7/LConn1
  Rigid Transform7/RConn1 -- Planar Joint/LConn1 -- Transform Sensor/LConn1 -- 6-DOF Joint/LConn1
  6-DOF Joint/RConn2 -- PS-Simulink Converter/LConn1
  6-DOF Joint/RConn3 -- PS-Simulink Converter1/LConn1
  6-DOF Joint/RConn4 -- PS-Simulink Converter2/LConn1
  PS-Simulink Converter3/LConn1 -- Transform Sensor/RConn2

== system Model_turn/LIMB 1: Back LEFT ==
  TARGET X [DEG] : Inport
  TARGET Y [DEG] : Inport  Port=2
  BANG-BANG CONTROLLER : MATLAB Function  TreatAsAtomicUnit=on
  Constant : Constant  Value=PWM_max
  "DUTY CYCLE " : Scope  NumInputPorts=4
  Derivative : Derivative
  Derivative1 : Derivative
  Integrator : Integrator
  Integrator1 : Integrator
  Limb 1 : Subsystem
      settings: PortSchema="{\"entries\":[{\"content\":{\"sides\":[{\"content\":{\"connectorIds\":[\"In1\",\"In2\",\"In3\",\"In4\"]},\"type\":\"ConnectorPlacement.EquallySpacedRectSide\",\"uuid\":\"1cfbebb6-90a9-4503-841a-11205e4f7b86\"},{\"content\":{\"connectorIds\":[\"Out1\",\"Out2\",\"Out3\",\"Out4\",\"Out5\",\"Out6\"],\"side\":\"RIGHT\"},\"type\":\"ConnectorPlacement.EquallySpacedRectSide\",\"uuid\":\"1fe5f3cc-98d4-4c2f-97d4-d32079cd1e1f\"},{\"content\":{\"connectorIds\":[\"LConn1\"],\"side\":\"TOP\"},\"type\":\"ConnectorPlacement.EquallySpacedRectSide\",\"uuid\":\"8adc0629-c4c5-41e3-bf7c-2c474717e53c\"}]},\"type\":\"ConnectorPlacement.EquallySpacedConnector\",\"uuid\":\"10590026-c19e-4697-bf09-c537692c54fc\"}],\"packageUris\":[\"http://schema.mathworks.com/mf0/Connector/R2020b\"],\"version\":\"1.0\"}"
  PID CONTROLLER : MATLAB Function  TreatAsAtomicUnit=on
  POSITION : Scope  NumInputPorts=2
  Scope : Scope
  Sum : Sum  Inputs=|+-
  Sum1 : Sum  Inputs=|+-
  [0, 1]{,1..3} (4 alike) : Saturate  UpperLimit=1  LowerLimit=0
  Base1 : PMIOPort  Side=Left
  wires:
  PID CONTROLLER/4(D4) -> ?
  PID CONTROLLER/2(D2) -> ?
  "[0, 1]2"/1 -> Limb 1/2(Duty Cycle 3), "DUTY CYCLE "/3
  PID CONTROLLER/3(D3) -> ?
  Derivative/1 -> PID CONTROLLER/2(deX)
  TARGET X [DEG]/1 -> Sum1/1, BANG-BANG CONTROLLER/3(Target_X)
  PID CONTROLLER/1(D1) -> ?
  Integrator/1 -> PID CONTROLLER/3(seX)
  TARGET Y [DEG]/1 -> BANG-BANG CONTROLLER/4(Target_Y), Sum/1
  Sum/1 -> PID CONTROLLER/4(eY), Derivative1/1, Integrator1/1
  BANG-BANG CONTROLLER/2(D2) -> "[0, 1]1"/1
  Limb 1/1(theta_X) -> POSITION/1, Sum1/2, BANG-BANG CONTROLLER/1(theta_X)
  BANG-BANG CONTROLLER/1(D1) -> "[0, 1]"/1
  "[0, 1]"/1 -> "DUTY CYCLE "/1, Limb 1/4(Duty Cycle 1)
  Derivative1/1 -> PID CONTROLLER/5(deY)
  BANG-BANG CONTROLLER/4(D4) -> "[0, 1]3"/1
  Integrator1/1 -> PID CONTROLLER/6(seY)
  Constant/1 -> BANG-BANG CONTROLLER/5(PWM_max), PID CONTROLLER/7(PWM_max)
  "[0, 1]1"/1 -> "DUTY CYCLE "/2, Limb 1/3(Duty Cycle 2)
  Sum1/1 -> PID CONTROLLER/1(eX), Scope/1, Derivative/1, Integrator/1
  "[0, 1]3"/1 -> "DUTY CYCLE "/4, Limb 1/1(Duty Cycle 4)
  BANG-BANG CONTROLLER/3(D3) -> "[0, 1]2"/1
  Limb 1/2(theta_Y) -> POSITION/2, Sum/2, BANG-BANG CONTROLLER/2(theta_Y)
  connections:
  Base1/RConn1 -- Limb 1/LConn1

== system Model_turn/LIMB 1: Back RIGHT ==
  TARGET X [DEG] : Inport
  TARGET Y [DEG] : Inport  Port=2
  BANG-BANG CONTROLLER : MATLAB Function  TreatAsAtomicUnit=on
  Constant : Constant  Value=PWM_max
  "DUTY CYCLE " : Scope  NumInputPorts=4
  Derivative : Derivative
  Derivative1 : Derivative
  Integrator : Integrator
  Integrator1 : Integrator
  Limb 1 : Subsystem
      settings: PortSchema="{\"entries\":[{\"content\":{\"sides\":[{\"content\":{\"connectorIds\":[\"In1\",\"In2\",\"In3\",\"In4\"]},\"type\":\"ConnectorPlacement.EquallySpacedRectSide\",\"uuid\":\"1cfbebb6-90a9-4503-841a-11205e4f7b86\"},{\"content\":{\"connectorIds\":[\"Out1\",\"Out2\",\"Out3\",\"Out4\",\"Out5\",\"Out6\"],\"side\":\"RIGHT\"},\"type\":\"ConnectorPlacement.EquallySpacedRectSide\",\"uuid\":\"1fe5f3cc-98d4-4c2f-97d4-d32079cd1e1f\"},{\"content\":{\"connectorIds\":[\"LConn1\"],\"side\":\"TOP\"},\"type\":\"ConnectorPlacement.EquallySpacedRectSide\",\"uuid\":\"8adc0629-c4c5-41e3-bf7c-2c474717e53c\"}]},\"type\":\"ConnectorPlacement.EquallySpacedConnector\",\"uuid\":\"10590026-c19e-4697-bf09-c537692c54fc\"}],\"packageUris\":[\"http://schema.mathworks.com/mf0/Connector/R2020b\"],\"version\":\"1.0\"}"
  PID CONTROLLER : MATLAB Function  TreatAsAtomicUnit=on
  POSITION : Scope  NumInputPorts=2
  Scope : Scope
  Sum : Sum  Inputs=|+-
  Sum1 : Sum  Inputs=|+-
  [0, 1]{,1..3} (4 alike) : Saturate  UpperLimit=1  LowerLimit=0
  Base1 : PMIOPort  Side=Left
  wires:
  Limb 1/2(theta_Y) -> BANG-BANG CONTROLLER/2(theta_Y), Sum/2, POSITION/2
  BANG-BANG CONTROLLER/3(D3) -> "[0, 1]2"/1
  "[0, 1]3"/1 -> Limb 1/1(Duty Cycle 4), "DUTY CYCLE "/4
  Sum1/1 -> Integrator/1, Derivative/1, Scope/1, PID CONTROLLER/1(eX)
  "[0, 1]1"/1 -> Limb 1/3(Duty Cycle 2), "DUTY CYCLE "/2
  Constant/1 -> PID CONTROLLER/7(PWM_max), BANG-BANG CONTROLLER/5(PWM_max)
  Integrator1/1 -> PID CONTROLLER/6(seY)
  BANG-BANG CONTROLLER/4(D4) -> "[0, 1]3"/1
  Derivative1/1 -> PID CONTROLLER/5(deY)
  "[0, 1]"/1 -> Limb 1/4(Duty Cycle 1), "DUTY CYCLE "/1
  BANG-BANG CONTROLLER/1(D1) -> "[0, 1]"/1
  Limb 1/1(theta_X) -> BANG-BANG CONTROLLER/1(theta_X), Sum1/2, POSITION/1
  BANG-BANG CONTROLLER/2(D2) -> "[0, 1]1"/1
  Sum/1 -> Integrator1/1, Derivative1/1, PID CONTROLLER/4(eY)
  TARGET Y [DEG]/1 -> Sum/1, BANG-BANG CONTROLLER/4(Target_Y)
  Integrator/1 -> PID CONTROLLER/3(seX)
  PID CONTROLLER/1(D1) -> ?
  TARGET X [DEG]/1 -> BANG-BANG CONTROLLER/3(Target_X), Sum1/1
  Derivative/1 -> PID CONTROLLER/2(deX)
  PID CONTROLLER/3(D3) -> ?
  "[0, 1]2"/1 -> "DUTY CYCLE "/3, Limb 1/2(Duty Cycle 3)
  PID CONTROLLER/2(D2) -> ?
  PID CONTROLLER/4(D4) -> ?
  connections:
  Base1/RConn1 -- Limb 1/LConn1

== system Model_turn/LIMB 1: Center LEFT ==
  TARGET X [DEG] : Inport
  TARGET Y [DEG] : Inport  Port=2
  BANG-BANG CONTROLLER : MATLAB Function  TreatAsAtomicUnit=on
  Constant : Constant  Value=PWM_max
  "DUTY CYCLE " : Scope  NumInputPorts=4
  Derivative : Derivative
  Derivative1 : Derivative
  Integrator : Integrator
  Integrator1 : Integrator
  Limb 1 : Subsystem
      settings: PortSchema="{\"entries\":[{\"content\":{\"sides\":[{\"content\":{\"connectorIds\":[\"In1\",\"In2\",\"In3\",\"In4\"]},\"type\":\"ConnectorPlacement.EquallySpacedRectSide\",\"uuid\":\"1cfbebb6-90a9-4503-841a-11205e4f7b86\"},{\"content\":{\"connectorIds\":[\"Out1\",\"Out2\",\"Out3\",\"Out4\",\"Out5\",\"Out6\"],\"side\":\"RIGHT\"},\"type\":\"ConnectorPlacement.EquallySpacedRectSide\",\"uuid\":\"1fe5f3cc-98d4-4c2f-97d4-d32079cd1e1f\"},{\"content\":{\"connectorIds\":[\"LConn1\"],\"side\":\"TOP\"},\"type\":\"ConnectorPlacement.EquallySpacedRectSide\",\"uuid\":\"8adc0629-c4c5-41e3-bf7c-2c474717e53c\"}]},\"type\":\"ConnectorPlacement.EquallySpacedConnector\",\"uuid\":\"10590026-c19e-4697-bf09-c537692c54fc\"}],\"packageUris\":[\"http://schema.mathworks.com/mf0/Connector/R2020b\"],\"version\":\"1.0\"}"
  PID CONTROLLER : MATLAB Function  TreatAsAtomicUnit=on
  POSITION : Scope  NumInputPorts=2
  Scope : Scope
  Scope1 : Scope
  Sum : Sum  Inputs=|+-
  Sum1 : Sum  Inputs=|+-
  [0, 1]{,1..3} (4 alike) : Saturate  UpperLimit=1  LowerLimit=0
  Base1 : PMIOPort  Side=Left
  wires:
  Limb 1/2(theta_Y) -> BANG-BANG CONTROLLER/2(theta_Y), Sum/2, POSITION/2
  BANG-BANG CONTROLLER/3(D3) -> "[0, 1]2"/1
  "[0, 1]3"/1 -> Limb 1/1(Duty Cycle 4), "DUTY CYCLE "/4
  Sum1/1 -> Integrator/1, Derivative/1, Scope/1, PID CONTROLLER/1(eX)
  "[0, 1]1"/1 -> Limb 1/3(Duty Cycle 2), "DUTY CYCLE "/2
  Constant/1 -> PID CONTROLLER/7(PWM_max), BANG-BANG CONTROLLER/5(PWM_max)
  Integrator1/1 -> PID CONTROLLER/6(seY)
  BANG-BANG CONTROLLER/4(D4) -> "[0, 1]3"/1
  Derivative1/1 -> PID CONTROLLER/5(deY)
  "[0, 1]"/1 -> Limb 1/4(Duty Cycle 1), "DUTY CYCLE "/1
  BANG-BANG CONTROLLER/1(D1) -> "[0, 1]"/1
  Limb 1/1(theta_X) -> BANG-BANG CONTROLLER/1(theta_X), Sum1/2, POSITION/1
  BANG-BANG CONTROLLER/2(D2) -> "[0, 1]1"/1
  Sum/1 -> Integrator1/1, Derivative1/1, PID CONTROLLER/4(eY)
  TARGET Y [DEG]/1 -> Scope1/1, Sum/1, BANG-BANG CONTROLLER/4(Target_Y)
  Integrator/1 -> PID CONTROLLER/3(seX)
  PID CONTROLLER/1(D1) -> ?
  TARGET X [DEG]/1 -> BANG-BANG CONTROLLER/3(Target_X), Sum1/1
  Derivative/1 -> PID CONTROLLER/2(deX)
  PID CONTROLLER/3(D3) -> ?
  "[0, 1]2"/1 -> "DUTY CYCLE "/3, Limb 1/2(Duty Cycle 3)
  PID CONTROLLER/2(D2) -> ?
  PID CONTROLLER/4(D4) -> ?
  connections:
  Base1/RConn1 -- Limb 1/LConn1

== system Model_turn/LIMB 1: Center RIGHT ==
  TARGET X [DEG] : Inport
  TARGET Y [DEG] : Inport  Port=2
  BANG-BANG CONTROLLER : MATLAB Function  TreatAsAtomicUnit=on
  Constant : Constant  Value=PWM_max
  "DUTY CYCLE " : Scope  NumInputPorts=4
  Derivative : Derivative
  Derivative1 : Derivative
  Integrator : Integrator
  Integrator1 : Integrator
  Limb 1 : Subsystem
      settings: PortSchema="{\"entries\":[{\"content\":{\"sides\":[{\"content\":{\"connectorIds\":[\"In1\",\"In2\",\"In3\",\"In4\"]},\"type\":\"ConnectorPlacement.EquallySpacedRectSide\",\"uuid\":\"1cfbebb6-90a9-4503-841a-11205e4f7b86\"},{\"content\":{\"connectorIds\":[\"Out1\",\"Out2\",\"Out3\",\"Out4\",\"Out5\",\"Out6\"],\"side\":\"RIGHT\"},\"type\":\"ConnectorPlacement.EquallySpacedRectSide\",\"uuid\":\"1fe5f3cc-98d4-4c2f-97d4-d32079cd1e1f\"},{\"content\":{\"connectorIds\":[\"LConn1\"],\"side\":\"TOP\"},\"type\":\"ConnectorPlacement.EquallySpacedRectSide\",\"uuid\":\"8adc0629-c4c5-41e3-bf7c-2c474717e53c\"}]},\"type\":\"ConnectorPlacement.EquallySpacedConnector\",\"uuid\":\"10590026-c19e-4697-bf09-c537692c54fc\"}],\"packageUris\":[\"http://schema.mathworks.com/mf0/Connector/R2020b\"],\"version\":\"1.0\"}"
  PID CONTROLLER : MATLAB Function  TreatAsAtomicUnit=on
  POSITION : Scope  NumInputPorts=2
  Scope : Scope
  Sum : Sum  Inputs=|+-
  Sum1 : Sum  Inputs=|+-
  [0, 1]{,1..3} (4 alike) : Saturate  UpperLimit=1  LowerLimit=0
  Base1 : PMIOPort  Side=Left
  wires:
  PID CONTROLLER/4(D4) -> ?
  PID CONTROLLER/2(D2) -> ?
  "[0, 1]2"/1 -> Limb 1/2(Duty Cycle 3), "DUTY CYCLE "/3
  PID CONTROLLER/3(D3) -> ?
  Derivative/1 -> PID CONTROLLER/2(deX)
  TARGET X [DEG]/1 -> Sum1/1, BANG-BANG CONTROLLER/3(Target_X)
  PID CONTROLLER/1(D1) -> ?
  Integrator/1 -> PID CONTROLLER/3(seX)
  TARGET Y [DEG]/1 -> BANG-BANG CONTROLLER/4(Target_Y), Sum/1
  Sum/1 -> PID CONTROLLER/4(eY), Derivative1/1, Integrator1/1
  BANG-BANG CONTROLLER/2(D2) -> "[0, 1]1"/1
  Limb 1/1(theta_X) -> POSITION/1, Sum1/2, BANG-BANG CONTROLLER/1(theta_X)
  BANG-BANG CONTROLLER/1(D1) -> "[0, 1]"/1
  "[0, 1]"/1 -> "DUTY CYCLE "/1, Limb 1/4(Duty Cycle 1)
  Derivative1/1 -> PID CONTROLLER/5(deY)
  BANG-BANG CONTROLLER/4(D4) -> "[0, 1]3"/1
  Integrator1/1 -> PID CONTROLLER/6(seY)
  Constant/1 -> BANG-BANG CONTROLLER/5(PWM_max), PID CONTROLLER/7(PWM_max)
  "[0, 1]1"/1 -> "DUTY CYCLE "/2, Limb 1/3(Duty Cycle 2)
  Sum1/1 -> PID CONTROLLER/1(eX), Scope/1, Derivative/1, Integrator/1
  "[0, 1]3"/1 -> "DUTY CYCLE "/4, Limb 1/1(Duty Cycle 4)
  BANG-BANG CONTROLLER/3(D3) -> "[0, 1]2"/1
  Limb 1/2(theta_Y) -> POSITION/2, Sum/2, BANG-BANG CONTROLLER/2(theta_Y)
  connections:
  Base1/RConn1 -- Limb 1/LConn1

== system Model_turn/LIMB 1: Front LEFT ==
  TARGET X [DEG] : Inport
  TARGET Y [DEG] : Inport  Port=2
  BANG-BANG CONTROLLER : MATLAB Function  TreatAsAtomicUnit=on
  Constant : Constant  Value=PWM_max
  "DUTY CYCLE " : Scope  NumInputPorts=4
  Derivative : Derivative
  Derivative1 : Derivative
  Integrator : Integrator
  Integrator1 : Integrator
  Limb 1 : Subsystem
      settings: PortSchema="{\"entries\":[{\"content\":{\"sides\":[{\"content\":{\"connectorIds\":[\"In1\",\"In2\",\"In3\",\"In4\"]},\"type\":\"ConnectorPlacement.EquallySpacedRectSide\",\"uuid\":\"1cfbebb6-90a9-4503-841a-11205e4f7b86\"},{\"content\":{\"connectorIds\":[\"Out1\",\"Out2\",\"Out3\",\"Out4\",\"Out5\",\"Out6\"],\"side\":\"RIGHT\"},\"type\":\"ConnectorPlacement.EquallySpacedRectSide\",\"uuid\":\"1fe5f3cc-98d4-4c2f-97d4-d32079cd1e1f\"},{\"content\":{\"connectorIds\":[\"LConn1\"],\"side\":\"TOP\"},\"type\":\"ConnectorPlacement.EquallySpacedRectSide\",\"uuid\":\"8adc0629-c4c5-41e3-bf7c-2c474717e53c\"}]},\"type\":\"ConnectorPlacement.EquallySpacedConnector\",\"uuid\":\"10590026-c19e-4697-bf09-c537692c54fc\"}],\"packageUris\":[\"http://schema.mathworks.com/mf0/Connector/R2020b\"],\"version\":\"1.0\"}"
  PID CONTROLLER : MATLAB Function  TreatAsAtomicUnit=on
  POSITION : Scope  NumInputPorts=2
  Scope : Scope
  Scope1 : Scope
  Sum : Sum  Inputs=|+-
  Sum1 : Sum  Inputs=|+-
  [0, 1]{,1..3} (4 alike) : Saturate  UpperLimit=1  LowerLimit=0
  Base1 : PMIOPort  Side=Left
  wires:
  PID CONTROLLER/4(D4) -> ?
  PID CONTROLLER/2(D2) -> ?
  "[0, 1]2"/1 -> Limb 1/2(Duty Cycle 3), "DUTY CYCLE "/3
  PID CONTROLLER/3(D3) -> ?
  Derivative/1 -> PID CONTROLLER/2(deX)
  TARGET X [DEG]/1 -> Sum1/1, BANG-BANG CONTROLLER/3(Target_X)
  PID CONTROLLER/1(D1) -> ?
  Integrator/1 -> PID CONTROLLER/3(seX)
  TARGET Y [DEG]/1 -> BANG-BANG CONTROLLER/4(Target_Y), Sum/1
  Sum/1 -> PID CONTROLLER/4(eY), Derivative1/1, Integrator1/1
  BANG-BANG CONTROLLER/2(D2) -> "[0, 1]1"/1
  Limb 1/1(theta_X) -> POSITION/1, Sum1/2, BANG-BANG CONTROLLER/1(theta_X)
  BANG-BANG CONTROLLER/1(D1) -> "[0, 1]"/1
  "[0, 1]"/1 -> "DUTY CYCLE "/1, Limb 1/4(Duty Cycle 1)
  Derivative1/1 -> PID CONTROLLER/5(deY)
  BANG-BANG CONTROLLER/4(D4) -> "[0, 1]3"/1
  Integrator1/1 -> PID CONTROLLER/6(seY)
  Constant/1 -> BANG-BANG CONTROLLER/5(PWM_max), PID CONTROLLER/7(PWM_max)
  "[0, 1]1"/1 -> "DUTY CYCLE "/2, Limb 1/3(Duty Cycle 2)
  Sum1/1 -> PID CONTROLLER/1(eX), Scope/1, Derivative/1, Integrator/1
  "[0, 1]3"/1 -> "DUTY CYCLE "/4, Limb 1/1(Duty Cycle 4)
  BANG-BANG CONTROLLER/3(D3) -> "[0, 1]2"/1
  Limb 1/2(theta_Y) -> POSITION/2, Sum/2, BANG-BANG CONTROLLER/2(theta_Y)
  Limb 1/4(GRF) -> Scope1/1
  connections:
  Base1/RConn1 -- Limb 1/LConn1

== system Model_turn/LIMB 1: Front RIGHT ==
  TARGET X [DEG] : Inport
  TARGET Y [DEG] : Inport  Port=2
  BANG-BANG CONTROLLER : MATLAB Function  TreatAsAtomicUnit=on
  Constant : Constant  Value=PWM_max
  "DUTY CYCLE " : Scope  NumInputPorts=4
  Derivative : Derivative
  Derivative1 : Derivative
  Integrator : Integrator
  Integrator1 : Integrator
  Limb 1 : Subsystem
      settings: PortSchema="{\"entries\":[{\"content\":{\"sides\":[{\"content\":{\"connectorIds\":[\"In1\",\"In2\",\"In3\",\"In4\"]},\"type\":\"ConnectorPlacement.EquallySpacedRectSide\",\"uuid\":\"1cfbebb6-90a9-4503-841a-11205e4f7b86\"},{\"content\":{\"connectorIds\":[\"Out1\",\"Out2\",\"Out3\",\"Out4\",\"Out5\",\"Out6\"],\"side\":\"RIGHT\"},\"type\":\"ConnectorPlacement.EquallySpacedRectSide\",\"uuid\":\"1fe5f3cc-98d4-4c2f-97d4-d32079cd1e1f\"},{\"content\":{\"connectorIds\":[\"LConn1\"],\"side\":\"TOP\"},\"type\":\"ConnectorPlacement.EquallySpacedRectSide\",\"uuid\":\"8adc0629-c4c5-41e3-bf7c-2c474717e53c\"}]},\"type\":\"ConnectorPlacement.EquallySpacedConnector\",\"uuid\":\"10590026-c19e-4697-bf09-c537692c54fc\"}],\"packageUris\":[\"http://schema.mathworks.com/mf0/Connector/R2020b\"],\"version\":\"1.0\"}"
  PID CONTROLLER : MATLAB Function  TreatAsAtomicUnit=on
  POSITION : Scope  NumInputPorts=2
  Scope : Scope
  Sum : Sum  Inputs=|+-
  Sum1 : Sum  Inputs=|+-
  [0, 1]{,1..3} (4 alike) : Saturate  UpperLimit=1  LowerLimit=0
  Base1 : PMIOPort  Side=Left
  wires:
  Limb 1/2(theta_Y) -> BANG-BANG CONTROLLER/2(theta_Y), Sum/2, POSITION/2
  BANG-BANG CONTROLLER/3(D3) -> "[0, 1]2"/1
  "[0, 1]3"/1 -> Limb 1/1(Duty Cycle 4), "DUTY CYCLE "/4
  Sum1/1 -> Integrator/1, Derivative/1, Scope/1, PID CONTROLLER/1(eX)
  "[0, 1]1"/1 -> Limb 1/3(Duty Cycle 2), "DUTY CYCLE "/2
  Constant/1 -> PID CONTROLLER/7(PWM_max), BANG-BANG CONTROLLER/5(PWM_max)
  Integrator1/1 -> PID CONTROLLER/6(seY)
  BANG-BANG CONTROLLER/4(D4) -> "[0, 1]3"/1
  Derivative1/1 -> PID CONTROLLER/5(deY)
  "[0, 1]"/1 -> Limb 1/4(Duty Cycle 1), "DUTY CYCLE "/1
  BANG-BANG CONTROLLER/1(D1) -> "[0, 1]"/1
  Limb 1/1(theta_X) -> BANG-BANG CONTROLLER/1(theta_X), Sum1/2, POSITION/1
  BANG-BANG CONTROLLER/2(D2) -> "[0, 1]1"/1
  Sum/1 -> Integrator1/1, Derivative1/1, PID CONTROLLER/4(eY)
  TARGET Y [DEG]/1 -> Sum/1, BANG-BANG CONTROLLER/4(Target_Y)
  Integrator/1 -> PID CONTROLLER/3(seX)
  PID CONTROLLER/1(D1) -> ?
  TARGET X [DEG]/1 -> BANG-BANG CONTROLLER/3(Target_X), Sum1/1
  Derivative/1 -> PID CONTROLLER/2(deX)
  PID CONTROLLER/3(D3) -> ?
  "[0, 1]2"/1 -> "DUTY CYCLE "/3, Limb 1/2(Duty Cycle 3)
  PID CONTROLLER/2(D2) -> ?
  PID CONTROLLER/4(D4) -> ?
  connections:
  Base1/RConn1 -- Limb 1/LConn1
